simulink library "csu_tts_thruster_time_safety_lib"  (R2015b)
settings: Solver=ode45  StartTime=0.0  StopTime=10.0  RelTol=1e-3
values from neighbouring files (symbols this model uses):
  act_full_on_duration = uint32( 120 )    [csc_act_actuator_manager_init.m]
undefined symbols (not defined in the file or in its folder): cac_acs_minimum_coarse_thruster_ontime
libraries: util_info_lib x1
settings Model: Creator=escrane  LastModifiedBy=jimkaidy
settings DataIOCC: SaveFormat=Array
settings DebuggingCC: UnderspecifiedInitializationDetection=Classic  MergeDetectMultiDrivingBlocksExec=none  SolverPrmCheckMsg=warning
settings HardwareCC: ProdBitPerPointer=32  ProdLargestAtomicFloat=None  ProdIntDivRoundTo=Undefined  ProdEndianess=Unspecified  ProdWordSize=32  ProdHWDeviceType=32-bit Generic
settings GRTTargetCC: GeneratePreprocessorConditionals=Disable all
settings ConfigComp: CovModelRefEnable=Off  CovSFcnEnable=off

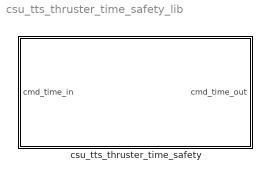
== system csu_tts_thruster_time_safety_lib ==
  csu_tts_thruster_time_safety : Subsystem

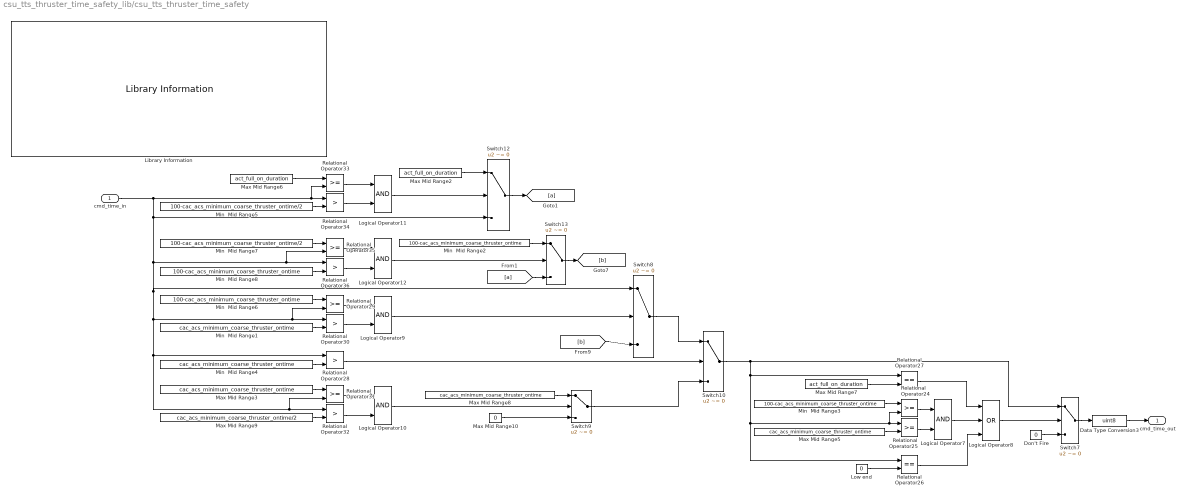
== system csu_tts_thruster_time_safety_lib/csu_tts_thruster_time_safety ==
  cmd_time_in : Inport
  Data Type Conversion3 : DataTypeConversion  OutDataTypeStr=uint8
  Don't Fire : Constant  Value=0
  Library Information : util_info_lib/Library Information  owner='NONE'
  Logical Operator{7,9..12} (5 alike) : Logic  AllPortsSameDT=off  OutDataTypeStr=boolean
  Logical Operator8 : Logic  Operator=OR  Inputs=3  AllPortsSameDT=off  OutDataTypeStr=boolean
  Low end : Constant  Value=0
  Max Mid Range10 : Constant  Value=0
  Max Mid Range2 : Constant  Value=act_full_on_duration
  Max Mid Range3 : Constant  Value=cac_acs_minimum_coarse_thruster_ontime
  Max Mid Range5 : Constant  Value=cac_acs_minimum_coarse_thruster_ontime
  Max Mid Range6 : Constant  Value=act_full_on_duration
  Max Mid Range7 : Constant  Value=act_full_on_duration
  Max Mid Range8 : Constant  Value=cac_acs_minimum_coarse_thruster_ontime
  Max Mid Range9 : Constant  Value=cac_acs_minimum_coarse_thruster_ontime/2
  Min  Mid Range1 : Constant  Value=cac_acs_minimum_coarse_thruster_ontime
  Min  Mid Range{2..3,6,8} (4 alike) : Constant  Value=100-cac_acs_minimum_coarse_thruster_ontime
  Min  Mid Range4 : Constant  Value=cac_acs_minimum_coarse_thruster_ontime
  Min  Mid Range5 : Constant  Value=100-cac_acs_minimum_coarse_thruster_ontime/2
  Min  Mid Range7 : Constant  Value=100-cac_acs_minimum_coarse_thruster_ontime/2
  Relational Operator{24..25,29,31,33,35} (6 alike) : RelationalOperator  OutDataTypeStr=boolean
  Relational Operator26 : RelationalOperator  Operator===  OutDataTypeStr=boolean
  Relational Operator27 : RelationalOperator  Operator===  OutDataTypeStr=boolean
  Relational Operator{28,30,32,34,36} (5 alike) : RelationalOperator  Operator=>  OutDataTypeStr=boolean
  Switch{7..10,12..13} (6 alike) : Switch  Criteria=u2 ~= 0
  cmd_time_out : Outport
  wires:
  cmd_time_in/1 -> Relational Operator33/2, Relational Operator34/1, Switch8/1, Relational Operator29/2, Relational Operator30/1, Relational Operator28/1, Relational Operator31/2, Relational Operator32/1, Relational Operator35/2, Relational Operator36/1, Switch12/3
  Switch7/1 -> Data Type Conversion3/1
  Max Mid Range10/1 -> Switch9/3
  Logical Operator12/1 -> Switch13/2
  Relational Operator36/1 -> Logical Operator12/2
  Relational Operator35/1 -> Logical Operator12/1
  Max Mid Range2/1 -> Switch12/1
  Logical Operator11/1 -> Switch12/2
  Relational Operator34/1 -> Logical Operator11/2
  Relational Operator33/1 -> Logical Operator11/1
  Min  Mid Range8/1 -> Relational Operator36/2
  Min  Mid Range7/1 -> Relational Operator35/1
  Min  Mid Range5/1 -> Relational Operator34/2
  Max Mid Range6/1 -> Relational Operator33/1
  Switch8/1 -> Switch10/1
  Relational Operator28/1 -> Switch10/2
  Min  Mid Range4/1 -> Relational Operator28/2
  Switch10/1 -> Relational Operator26/1, Relational Operator24/2, Relational Operator25/1, Relational Operator27/1, Switch7/1
  Switch9/1 -> Switch10/3
  Logical Operator9/1 -> Switch8/2
  Max Mid Range8/1 -> Switch9/1
  Logical Operator10/1 -> Switch9/2
  Relational Operator32/1 -> Logical Operator10/2
  Relational Operator31/1 -> Logical Operator10/1
  Max Mid Range9/1 -> Relational Operator32/2
  Max Mid Range3/1 -> Relational Operator31/1
  Relational Operator30/1 -> Logical Operator9/2
  Relational Operator29/1 -> Logical Operator9/1
  Min  Mid Range1/1 -> Relational Operator30/2
  Min  Mid Range6/1 -> Relational Operator29/1
  Don't Fire/1 -> Switch7/3
  Logical Operator8/1 -> Switch7/2
  Low end/1 -> Relational Operator26/2
  Relational Operator26/1 -> Logical Operator8/3
  Logical Operator7/1 -> Logical Operator8/2
  Relational Operator27/1 -> Logical Operator8/1
  Max Mid Range7/1 -> Relational Operator27/2
  Max Mid Range5/1 -> Relational Operator25/2
  Min  Mid Range3/1 -> Relational Operator24/1
  Relational Operator25/1 -> Logical Operator7/2
  Relational Operator24/1 -> Logical Operator7/1
  Data Type Conversion3/1 -> cmd_time_out/1
  Switch13/1 -> [b]
  [b] -> Switch8/3
  [a] -> Switch13/3
  Switch12/1 -> [a]
  Min  Mid Range2/1 -> Switch13/1
